simulink model "SiMappedEngine"  (R2017b)
settings: Solver=VariableStepAuto  StartTime=0.0  StopTime=inf  RelTol=1e-3  EnableMultiTasking=on
model workspace (MAT data in the model file):
  AccPwrbp = [0 1.5]
  AccSpdbp = [300 750]
  AfrStoich = 14.6
  Cps = 2
  NCyl = 4
  Pstd = 101325
  Rair = 287
  TimeCnstECP = 0.125
  TimeCnstEGR = 0.125
  TimeCnstETC = 0.085
  TimeCnstICP = 0.125
  TimeCnstIVL = 0.125
  TimeCnstMFA = 0.125
  TimeCnstSWVA = 0.125
  TimeCnstVCR = 0.125
  TimeCnstVGT = 0.15
  TimeCnstVIRL = 0.125
  TimeCnstWGA = 0.15
  Tstd = 293.15
  Vd = 0.0015
  f_air = [0 0 0 0 0 0 0 0 0 0 0 0 ... (256 elements, 16x16)]
  f_co = [0 0 0 0 0 0 0 0 0 0 0 0 ... (256 elements, 16x16)]
  f_co2 = [0 0 0 0 0 0 0 0 0 0 0 0 ... (256 elements, 16x16)]
  f_eff = [0 350.973137795 318.760126422 304.457775397 296.264860975 291.399796092 291.399634744 291.399447014 291.399182505 291.39897016 291.39870507 291.398494441 ... (256 elements, 16x16)]
  f_fuel = [0 0 0 0 0 0 0 0 0 0 0 0 ... (256 elements, 16x16)]
  f_hc = [0 0 0 0 0 0 0 0 0 0 0 0 ... (256 elements, 16x16)]
  f_nox = [0 0 0 0 0 0 0 0 0 0 0 0 ... (256 elements, 16x16)]
  f_pm = [0 0 0 0 0 0 0 0 0 0 0 0 ... (256 elements, 16x16)]
  f_tbrake = [0 33.5982453939 45.8470209066 56.5675272071 68.244809911 76.222788533 76.2227350264 76.2228412777 76.2230443728 76.2232177986 76.223431925 76.2235956457 ... (256 elements, 16x16)]
  f_tbrake_n_bpt = [0 750 1053.57142857 1357.14285714 1660.71428571 1964.28571429 2267.85714286 2571.42857143 2875 3178.57142857 3482.14285714 3785.71428571 ... (16 elements, 1x16)]
  f_tbrake_t_bpt = [0 15 26.4285714286 37.8571428571 49.2857142857 60.7142857143 72.1428571429 83.5714285714 95 106.428571429 117.857142857 129.285714286 ... (16 elements, 1x16)]
  f_texh = [767.640829797 767.64454905 788.103208022 800.869130868 880.777600935 909.697751416 909.697090822 909.697210127 909.697674873 909.698116175 909.698671892 909.699093491 ... (256 elements, 16x16)]
  f_twc_eff_co = [0.17 0.25 0.45 0.99 0.99 0.99 0.99]
  f_twc_eff_hc = [0.21 0.375 0.75 0.98 0.98 0.98 0.98]
  f_twc_eff_lam = [0.909090909 0.944055944 0.979020979 1 1.013986014 1.048951049 1.083916084]
  f_twc_eff_nox = [0.98 0.98 0.98 0.97 0.05 0.02 0]
libraries: autolibenginesystems x1
(part 2 of 2)

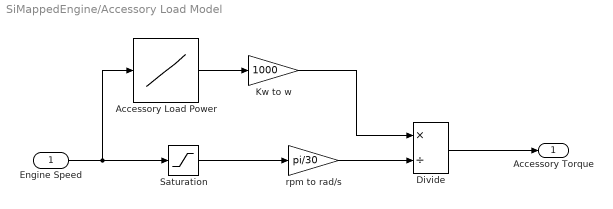
== system SiMappedEngine/Accessory Load Model ==
  Engine Speed : Inport
  Accessory Load Power : Lookup_n-D  NumberOfTableDimensions=1  LookupTableObject=''  BreakpointsForDimension1=AccSpdbp  Table=AccPwrbp  ExtrapMethod=Clip  InternalRulePriority=Speed  RndMeth=Simplest  InputSameDT=on
  Divide : Product  Inputs=*/
  Kw to w : Gain  Gain=1000
  Saturation : Saturate  UpperLimit=Inf  LowerLimit=300
  rpm to rad/s : Gain  Gain=pi/30
  Accessory Torque : Outport
  wires:
  Divide/1 -> Accessory Torque/1
  Accessory Load Power/1 -> Kw to w/1
  Engine Speed/1 -> Accessory Load Power/1, Saturation/1
  Saturation/1 -> rpm to rad/s/1
  rpm to rad/s/1 -> Divide/2
  Kw to w/1 -> Divide/1

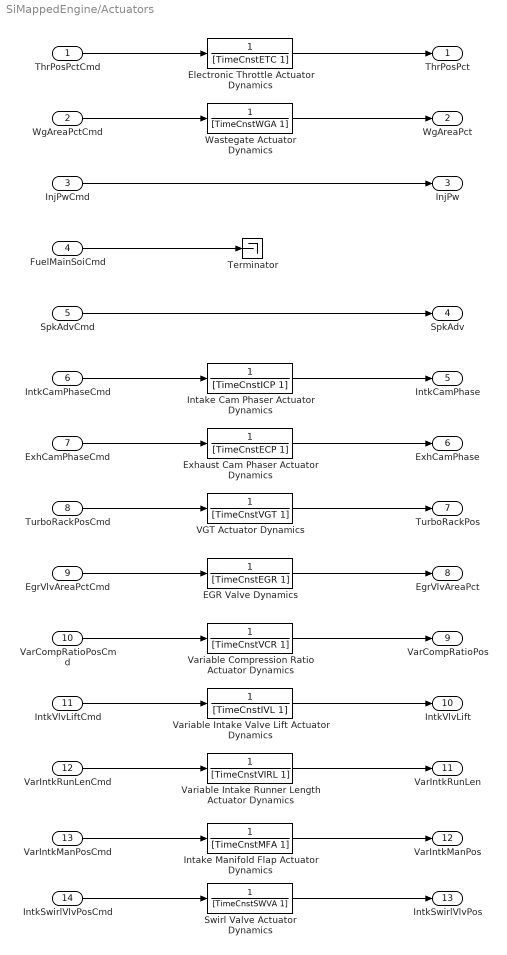
== system SiMappedEngine/Actuators ==
  ThrPosPctCmd : Inport  Unit=%
  WgAreaPctCmd : Inport  Port=2  Unit=%
  InjPwCmd : Inport  Port=3  Unit=ms
  FuelMainSoiCmd : Inport  Port=4  Unit=deg
  SpkAdvCmd : Inport  Port=5  Unit=deg
  IntkCamPhaseCmd : Inport  Port=6  Unit=deg
  ExhCamPhaseCmd : Inport  Port=7  Unit=deg
  TurboRackPosCmd : Inport  Port=8  Unit=1
  EgrVlvAreaPctCmd : Inport  Port=9  Unit=%
  VarCompRatioPosCmd : Inport  Port=10
  IntkVlvLiftCmd : Inport  Port=11
  VarIntkRunLenCmd : Inport  Port=12
  VarIntkManPosCmd : Inport  Port=13
  IntkSwirlVlvPosCmd : Inport  Port=14
  EGR Valve Dynamics : TransferFcn  Denominator=[TimeCnstEGR 1]
  Electronic Throttle Actuator Dynamics : TransferFcn  Denominator=[TimeCnstETC 1]
  Exhaust Cam Phaser Actuator Dynamics : TransferFcn  Denominator=[TimeCnstECP 1]
  Intake Cam Phaser Actuator Dynamics : TransferFcn  Denominator=[TimeCnstICP 1]
  Intake Manifold Flap Actuator Dynamics : TransferFcn  Denominator=[TimeCnstMFA 1]
  Swirl Valve Actuator Dynamics : TransferFcn  Denominator=[TimeCnstSWVA 1]
  Terminator : Terminator
  VGT Actuator Dynamics : TransferFcn  Denominator=[TimeCnstVGT 1]
  Variable Compression Ratio Actuator Dynamics : TransferFcn  Denominator=[TimeCnstVCR 1]
  Variable Intake Runner Length Actuator Dynamics : TransferFcn  Denominator=[TimeCnstVIRL 1]
  Variable Intake Valve Lift Actuator Dynamics : TransferFcn  Denominator=[TimeCnstIVL 1]
  Wastegate Actuator Dynamics : TransferFcn  Denominator=[TimeCnstWGA 1]
  ThrPosPct : Outport  Unit=%
  WgAreaPct : Outport  Port=2  Unit=%
  InjPw : Outport  Port=3
  SpkAdv : Outport  Port=4
  IntkCamPhase : Outport  Port=5  Unit=deg
  ExhCamPhase : Outport  Port=6  Unit=deg
  TurboRackPos : Outport  Port=7  Unit=1
  EgrVlvAreaPct : Outport  Port=8  Unit=%
  VarCompRatioPos : Outport  Port=9
  IntkVlvLift : Outport  Port=10
  VarIntkRunLen : Outport  Port=11
  VarIntkManPos : Outport  Port=12
  IntkSwirlVlvPos : Outport  Port=13
  wires:
  Variable Compression Ratio Actuator Dynamics/1 -> VarCompRatioPos/1
  Variable Intake Valve Lift Actuator Dynamics/1 -> IntkVlvLift/1
  Variable Intake Runner Length Actuator Dynamics/1 -> VarIntkRunLen/1
  Intake Manifold Flap Actuator Dynamics/1 -> VarIntkManPos/1
  Swirl Valve Actuator Dynamics/1 -> IntkSwirlVlvPos/1
  Intake Cam Phaser Actuator Dynamics/1 -> IntkCamPhase/1
  Exhaust Cam Phaser Actuator Dynamics/1 -> ExhCamPhase/1
  Wastegate Actuator Dynamics/1 -> WgAreaPct/1
  Electronic Throttle Actuator Dynamics/1 -> ThrPosPct/1
  FuelMainSoiCmd/1 -> Terminator/1
  IntkVlvLiftCmd/1 -> Variable Intake Valve Lift Actuator Dynamics/1
  IntkSwirlVlvPosCmd/1 -> Swirl Valve Actuator Dynamics/1
  WgAreaPctCmd/1 -> Wastegate Actuator Dynamics/1
  ThrPosPctCmd/1 -> Electronic Throttle Actuator Dynamics/1
  ExhCamPhaseCmd/1 -> Exhaust Cam Phaser Actuator Dynamics/1
  IntkCamPhaseCmd/1 -> Intake Cam Phaser Actuator Dynamics/1
  VarIntkManPosCmd/1 -> Intake Manifold Flap Actuator Dynamics/1
  VarCompRatioPosCmd/1 -> Variable Compression Ratio Actuator Dynamics/1
  VarIntkRunLenCmd/1 -> Variable Intake Runner Length Actuator Dynamics/1
  InjPwCmd/1 -> InjPw/1
  VGT Actuator Dynamics/1 -> TurboRackPos/1
  EGR Valve Dynamics/1 -> EgrVlvAreaPct/1
  TurboRackPosCmd/1 -> VGT Actuator Dynamics/1
  EgrVlvAreaPctCmd/1 -> EGR Valve Dynamics/1
  SpkAdvCmd/1 -> SpkAdv/1

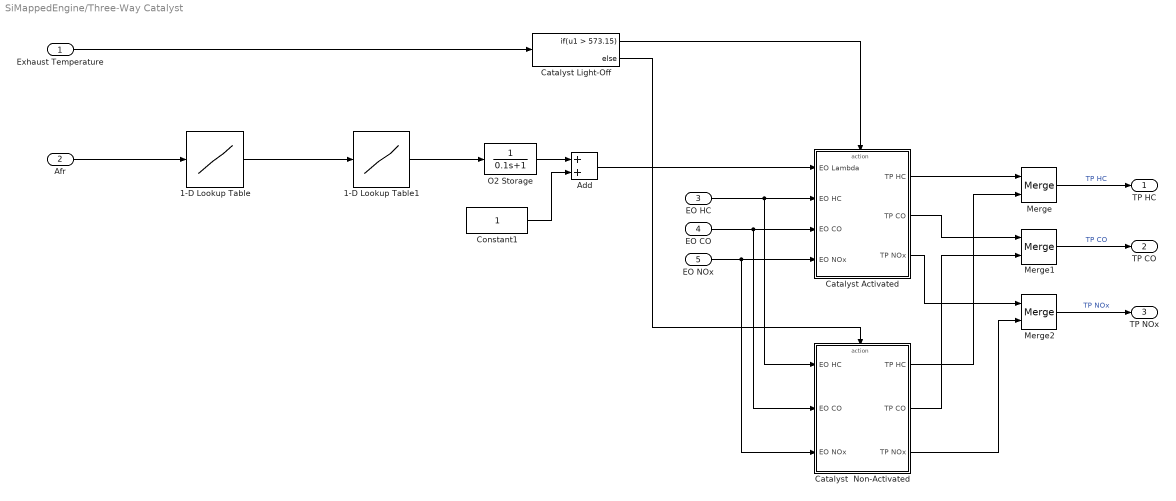
== system SiMappedEngine/Three-Way Catalyst ==
  Exhaust Temperature : Inport
  Afr : Inport  Port=2
  EO HC : Inport  Port=3
  EO CO : Inport  Port=4
  EO NOx : Inport  Port=5
  1-D Lookup Table : Lookup_n-D  NumberOfTableDimensions=1  BreakpointsForDimension1=[0 15 100]  Table=[0 15 AfrStoich]/AfrStoich  ExtrapMethod=Clip  InternalRulePriority=Speed  RndMeth=Simplest  InputSameDT=on
  1-D Lookup Table1 : Lookup_n-D  NumberOfTableDimensions=1  BreakpointsForDimension1=[0 0.97 1.03 1.1]  Table=[-1 0 0 0.07]  ExtrapMethod=Clip  InternalRulePriority=Speed  RndMeth=Simplest  InputSameDT=on
  Add : Sum
  Catalyst  Non-Activated : Subsystem
  Catalyst Activated : Subsystem
  Catalyst Light-Off : If  IfExpression=u1 > 573.15
  Constant1 : Constant
  Merge : Merge
  Merge1 : Merge
  Merge2 : Merge
  O2 Storage : TransferFcn  Denominator=[0.1 1]
  TP HC : Outport  Unit=kg/s
  TP CO : Outport  Port=2  Unit=kg/s
  TP NOx : Outport  Port=3  Unit=kg/s
  wires:
  EO HC/1 -> Catalyst  Non-Activated/1(EO HC), Catalyst Activated/2(EO HC)
  EO CO/1 -> Catalyst  Non-Activated/2(EO CO), Catalyst Activated/3(EO CO)
  EO NOx/1 -> Catalyst  Non-Activated/3(EO NOx), Catalyst Activated/4(EO NOx)
  Merge/1 -> TP HC/1  "TP HC"
  Merge1/1 -> TP CO/1  "TP CO"
  Merge2/1 -> TP NOx/1  "TP NOx"
  Catalyst Light-Off/1 -> Catalyst Activated/Action
  Catalyst Light-Off/2 -> Catalyst  Non-Activated/Action
  Exhaust Temperature/1 -> Catalyst Light-Off/1
  Catalyst Activated/1(TP HC) -> Merge/1
  Catalyst  Non-Activated/1(TP HC) -> Merge/2
  Catalyst Activated/2(TP CO) -> Merge1/1
  Catalyst  Non-Activated/2(TP CO) -> Merge1/2
  Catalyst Activated/3(TP NOx) -> Merge2/1
  Catalyst  Non-Activated/3(TP NOx) -> Merge2/2
  1-D Lookup Table1/1 -> O2 Storage/1
  Constant1/1 -> Add/2
  O2 Storage/1 -> Add/1
  Add/1 -> Catalyst Activated/1(EO Lambda)
  1-D Lookup Table/1 -> 1-D Lookup Table1/1
  Afr/1 -> 1-D Lookup Table/1

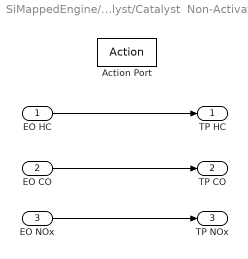
== system SiMappedEngine/Three-Way Catalyst/Catalyst  Non-Activated ==
  EO HC : Inport
  EO CO : Inport  Port=2
  EO NOx : Inport  Port=3
  Action Port : ActionPort  ActionType=else
  TP HC : Outport
  TP CO : Outport  Port=2
  TP NOx : Outport  Port=3
  wires:
  EO HC/1 -> TP HC/1
  EO CO/1 -> TP CO/1
  EO NOx/1 -> TP NOx/1

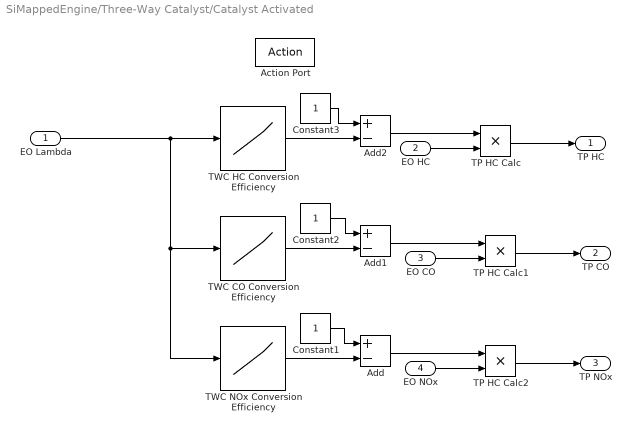
== system SiMappedEngine/Three-Way Catalyst/Catalyst Activated ==
  EO Lambda : Inport
  EO HC : Inport  Port=2
  EO CO : Inport  Port=3
  EO NOx : Inport  Port=4
  Action Port : ActionPort  ActionType=then
  Add : Sum  Inputs=+-
  Add1 : Sum  Inputs=+-
  Add2 : Sum  Inputs=+-
  Constant1 : Constant
  Constant2 : Constant
  Constant3 : Constant
  TP HC Calc : Product  Inputs=**
  TP HC Calc1 : Product  Inputs=**
  TP HC Calc2 : Product  Inputs=**
  TWC CO Conversion Efficiency : Lookup_n-D  NumberOfTableDimensions=1  LookupTableObject=''  BreakpointsForDimension1=f_twc_eff_lam  Table=f_twc_eff_co  ExtrapMethod=Clip  InternalRulePriority=Speed  RndMeth=Simplest  InputSameDT=on
  TWC HC Conversion Efficiency : Lookup_n-D  NumberOfTableDimensions=1  LookupTableObject=''  BreakpointsForDimension1=f_twc_eff_lam  Table=f_twc_eff_hc  ExtrapMethod=Clip  InternalRulePriority=Speed  RndMeth=Simplest  InputSameDT=on
  TWC NOx Conversion Efficiency : Lookup_n-D  NumberOfTableDimensions=1  LookupTableObject=''  BreakpointsForDimension1=f_twc_eff_lam  Table=f_twc_eff_nox  ExtrapMethod=Clip  InternalRulePriority=Speed  RndMeth=Simplest  InputSameDT=on
  TP HC : Outport
  TP CO : Outport  Port=2
  TP NOx : Outport  Port=3
  wires:
  EO HC/1 -> TP HC Calc/2
  TP HC Calc/1 -> TP HC/1
  Add/1 -> TP HC Calc2/1
  Constant1/1 -> Add/1
  TP HC Calc1/1 -> TP CO/1
  TWC HC Conversion Efficiency/1 -> Add2/2
  Add1/1 -> TP HC Calc1/1
  EO CO/1 -> TP HC Calc1/2
  TWC NOx Conversion Efficiency/1 -> Add/2
  TP HC Calc2/1 -> TP NOx/1
  EO NOx/1 -> TP HC Calc2/2
  EO Lambda/1 -> TWC NOx Conversion Efficiency/1, TWC CO Conversion Efficiency/1, TWC HC Conversion Efficiency/1
  Constant2/1 -> Add1/1
  TWC CO Conversion Efficiency/1 -> Add1/2
  Constant3/1 -> Add2/1
  Add2/1 -> TP HC Calc/1
